simulink model "Task3"  (R2013b)
settings: Solver=ode45  StartTime=0.0  StopTime=1  RelTol=1e-3
settings Model: Creator=barnetdavi  LastModifiedBy=barnetdavi

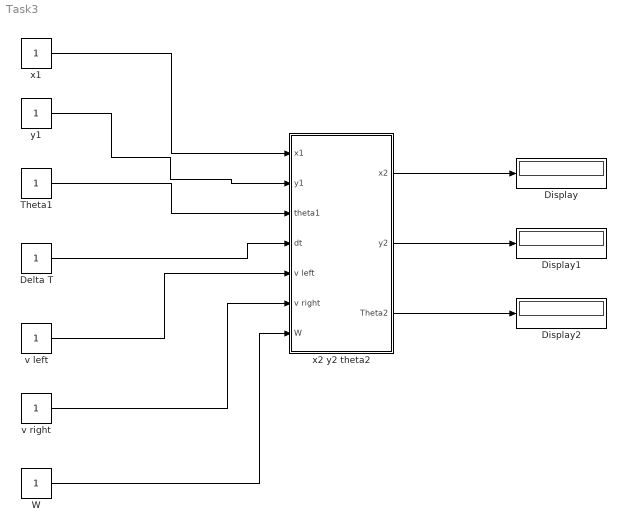
== system Task3 ==
  Delta T : Constant
  Display : Display
  Display1 : Display
  Display2 : Display
  Theta1 : Constant
  W : Constant
  v left : Constant
  v right : Constant
  x1 : Constant
  x2 y2 theta2 : Subsystem
  y1 : Constant
  wires:
  x1/1 -> x2 y2 theta2/1(x1)
  y1/1 -> x2 y2 theta2/2(y1)
  Theta1/1 -> x2 y2 theta2/3(theta1)
  Delta T/1 -> x2 y2 theta2/4(dt)
  v left/1 -> x2 y2 theta2/5(v left)
  v right/1 -> x2 y2 theta2/6(v right)
  W/1 -> x2 y2 theta2/7(W)
  x2 y2 theta2/1(x2) -> Display/1
  x2 y2 theta2/2(y2) -> Display1/1
  x2 y2 theta2/3(Theta2) -> Display2/1

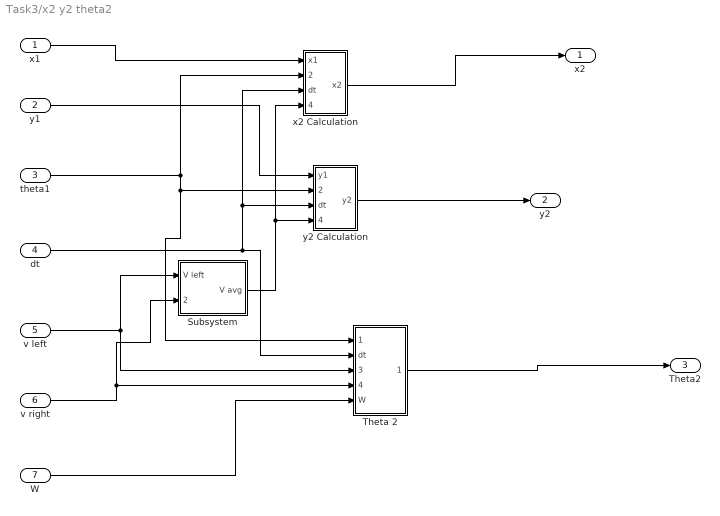
== system Task3/x2 y2 theta2 ==
  x1 : Inport
  y1 : Inport  Port=2
  theta1 : Inport  Port=3
  dt : Inport  Port=4
  v left : Inport  Port=5
  v right : Inport  Port=6
  W : Inport  Port=7
  Subsystem : Subsystem
  "Theta 2 " : Subsystem
  x2 Calculation : Subsystem
  y2 Calculation : Subsystem
  x2 : Outport
  y2 : Outport  Port=2
  Theta2 : Outport  Port=3
  wires:
  v left/1 -> "Theta 2 "/3(v left), Subsystem/1(V left)
  v right/1 -> Subsystem/2(V right), "Theta 2 "/4(v right)
  x1/1 -> x2 Calculation/1(x1)
  W/1 -> "Theta 2 "/5(W)
  "Theta 2 "/1(Out1) -> Theta2/1
  dt/1 -> "Theta 2 "/2(dt), y2 Calculation/3(dt), x2 Calculation/3(dt)
  x2 Calculation/1(x2) -> x2/1
  y2 Calculation/1(y2) -> y2/1
  theta1/1 -> x2 Calculation/2(theta1), "Theta 2 "/1(Theta 1), y2 Calculation/2(theta1)
  y1/1 -> y2 Calculation/1(y1)
  Subsystem/1(V avg) -> y2 Calculation/4(V avg), x2 Calculation/4(V avg)

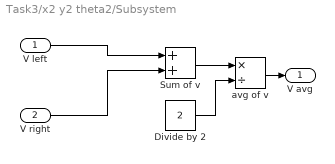
== system Task3/x2 y2 theta2/Subsystem ==
  V left : Inport
  V right : Inport  Port=2
  Divide by 2 : Constant  Value=2
  Sum of v : Sum
  avg of v : Product  Inputs=*/
  V avg : Outport
  wires:
  Divide by 2/1 -> avg of v/2
  avg of v/1 -> V avg/1
  Sum of v/1 -> avg of v/1
  V right/1 -> Sum of v/2
  V left/1 -> Sum of v/1

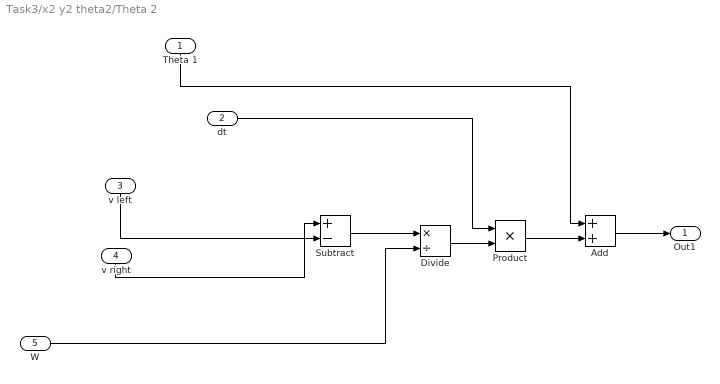
== system Task3/x2 y2 theta2/Theta 2  ==
  Theta 1 : Inport
  dt : Inport  Port=2
  v left : Inport  Port=3
  v right : Inport  Port=4
  W : Inport  Port=5
  Add : Sum
  Divide : Product  Inputs=*/
  Product : Product
  Subtract : Sum  Inputs=+-
  Out1 : Outport
  wires:
  Theta 1/1 -> Add/1
  Product/1 -> Add/2
  Divide/1 -> Product/2
  v left/1 -> Subtract/2
  v right/1 -> Subtract/1
  dt/1 -> Product/1
  Add/1 -> Out1/1
  Subtract/1 -> Divide/1
  W/1 -> Divide/2

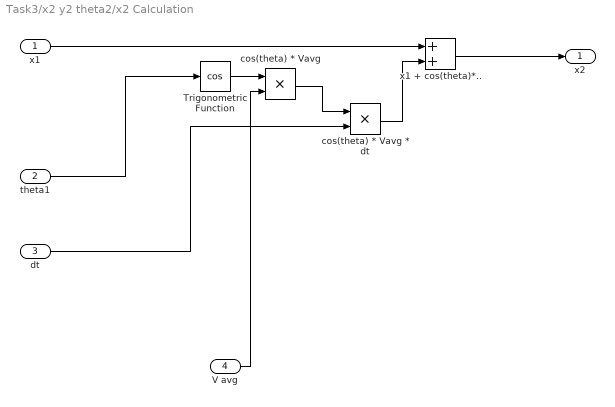
== system Task3/x2 y2 theta2/x2 Calculation ==
  x1 : Inport
  theta1 : Inport  Port=2
  dt : Inport  Port=3
  V avg : Inport  Port=4
  Trigonometric Function : Trigonometry  Operator=cos
  cos(theta) * Vavg : Product
  cos(theta) * Vavg * dt : Product
  x1 + cos(theta)*.. : Sum
  x2 : Outport
  wires:
  V avg/1 -> cos(theta) * Vavg/2
  x1/1 -> x1 + cos(theta)*../1
  Trigonometric Function/1 -> cos(theta) * Vavg/1
  dt/1 -> cos(theta) * Vavg * dt/2
  x1 + cos(theta)*../1 -> x2/1
  theta1/1 -> Trigonometric Function/1
  cos(theta) * Vavg/1 -> cos(theta) * Vavg * dt/1
  cos(theta) * Vavg * dt/1 -> x1 + cos(theta)*../2

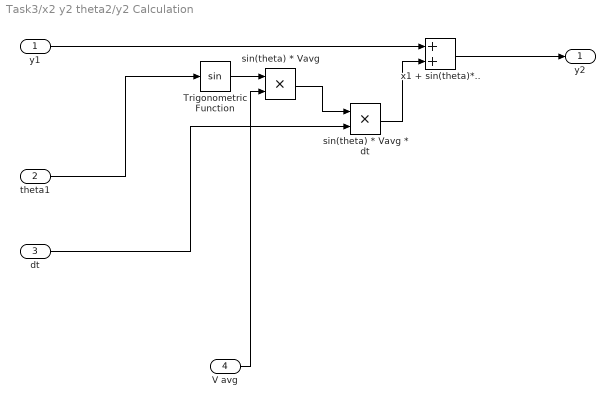
== system Task3/x2 y2 theta2/y2 Calculation ==
  y1 : Inport
  theta1 : Inport  Port=2
  dt : Inport  Port=3
  V avg : Inport  Port=4
  Trigonometric Function : Trigonometry
  sin(theta) * Vavg : Product
  sin(theta) * Vavg * dt : Product
  x1 + sin(theta)*.. : Sum
  y2 : Outport
  wires:
  V avg/1 -> sin(theta) * Vavg/2
  y1/1 -> x1 + sin(theta)*../1
  Trigonometric Function/1 -> sin(theta) * Vavg/1
  dt/1 -> sin(theta) * Vavg * dt/2
  x1 + sin(theta)*../1 -> y2/1
  theta1/1 -> Trigonometric Function/1
  sin(theta) * Vavg/1 -> sin(theta) * Vavg * dt/1
  sin(theta) * Vavg * dt/1 -> x1 + sin(theta)*../2
